simulink model "Final_project_template_R2020a_pt3 (1)"  (R2020a)
settings: Solver=FixedStepDiscrete  StartTime=0.0  StopTime=10.0  FixedStep=0.0005  RelTol=1e-3  EnableMultiTasking=on
InitFcn:
  | mbd_s32k_consistency_checks(bdroot(gcs));
values from neighbouring files (symbols this model uses):
  Ak = 100    [parameters_template (1).m]
  b = 100    [parameters_template (1).m]
  base_ids = [10, 20, 30, 40, 50, 70]    [parameters_template (1).m]
  dT = 0.01    [parameters_template (1).m]
  H = 20    [parameters_template (1).m]
  L1 = 1.6    [parameters_template (1).m]
  L2 = 0.8    [parameters_template (1).m]
  m = 2000    [parameters_template (1).m]
  n_desired = 2    [parameters_template (1).m]
  pot_gain = 1    [parameters_template (1).m]
  pot_offset = 512    [parameters_template (1).m]
  R = 1/5    (= 0.2)    [parameters_template (1).m]
  S_Kd1 = 0.03    [parameters_template (1).m]
  S_Kd2 = 25    [parameters_template (1).m]
  S_Kp1 = 0.45    [parameters_template (1).m]
  S_Kp2 = 1000    [parameters_template (1).m]
  V_Ki = 50    [parameters_template (1).m]
  V_Kp = 5000    [parameters_template (1).m]
undefined symbols (not defined in the file or in its folder): DiscIntNeverNeededParam, LQFP
libraries: mbd_s32k1xx_ec_toolbox x42, xpcutilitieslib x15, Veh_Sim x9, simulink x5
(part 2 of 2)

== system Final_project_template_R2020a_pt3 (1)/High Level Design/Outputs/Extract x,y,psi (Cars 1 - 6) ==
  s,n,psi,us (Cars 1 - 6) : Inport
  Demux : Demux  Outputs=6
  Extract x,y,psi : Subsystem
  Extract x,y,psi1 : Subsystem
  Extract x,y,psi2 : Subsystem
  Extract x,y,psi3 : Subsystem
  Extract x,y,psi4 : Subsystem
  Extract x,y,psi5 : Subsystem
  Mux : Mux  Inputs=6
  x,y,psi (Cars 1 - 6) : Outport  VectorParamsAs1DForOutWhenUnconnected=off
  wires:
  Demux/1 -> Extract x,y,psi/1(s,n,psi,us)
  Extract x,y,psi/1(x,y,psi) -> Mux/1
  Demux/2 -> Extract x,y,psi1/1(s,n,psi,us)
  Extract x,y,psi1/1(x,y,psi) -> Mux/2
  Demux/3 -> Extract x,y,psi2/1(s,n,psi,us)
  Extract x,y,psi2/1(x,y,psi) -> Mux/3
  Extract x,y,psi3/1(x,y,psi) -> Mux/4
  Demux/5 -> Extract x,y,psi4/1(s,n,psi,us)
  Extract x,y,psi4/1(x,y,psi) -> Mux/5
  s,n,psi,us (Cars 1 - 6)/1 -> Demux/1
  Extract x,y,psi5/1(x,y,psi) -> Mux/6
  Demux/6 -> Extract x,y,psi5/1(s,n,psi,us)
  Mux/1 -> x,y,psi (Cars 1 - 6)/1
  Demux/4 -> Extract x,y,psi3/1(s,n,psi,us)

== system Final_project_template_R2020a_pt3 (1)/High Level Design/Outputs/Tx CAN ==
  note: Use pack block to generate data arrays
      | Do not use any mailbox buffers that are used for receives
  note: Use FCAN_Send block to transmit two messages to the CAN bus
  s,n,psi,us : Inport
  "Byte Packing " : xpcutilitieslib/Byte Packing   MaskPackedDataType=uint8  MaskUnpackedDataTypes={'single'}  MaskAlignment=1
  Byte Packing 1 : xpcutilitieslib/Byte Packing   MaskPackedDataType=uint8  MaskUnpackedDataTypes={'single'}  MaskAlignment=1
  Constant : Constant  Value=8  OutDataTypeStr=uint8
  Constant1 : Constant  Value=8  OutDataTypeStr=uint8
  Demux : Demux  Outputs=2
  FCAN_Send : mbd_s32k1xx_ec_toolbox/Communication Blocks/CAN Blocks/FCAN_Send  can_instance=0  can_mode=Non-blocking  can_timeout_ms=0  can_mb_idx=0  can_extended_id=on  can_is_remote=off  can_id=41  show_adv_opts=off  can_fd_enable=off  can_enable_brs=off  can_fd_padding=0
  FCAN_Send1 : mbd_s32k1xx_ec_toolbox/Communication Blocks/CAN Blocks/FCAN_Send  can_instance=0  can_mode=Non-blocking  can_timeout_ms=0  can_mb_idx=1  can_extended_id=on  can_is_remote=off  can_id=42  show_adv_opts=off  can_fd_enable=off  can_enable_brs=off  can_fd_padding=0
  wires:
  s,n,psi,us/1 -> Demux/1
  Demux/1 -> "Byte Packing "/1
  Demux/2 -> Byte Packing 1/1
  "Byte Packing "/1 -> FCAN_Send/1
  Byte Packing 1/1 -> FCAN_Send1/1
  Constant1/1 -> FCAN_Send1/2
  Constant/1 -> FCAN_Send/2

== system Final_project_template_R2020a_pt3 (1)/High Level Design/Outputs/write torque ==
  Reaction Torque : Inport
  reaction torque : Subsystem
  wires:
  Reaction Torque/1 -> reaction torque/1(torque)

== system Final_project_template_R2020a_pt3 (1)/High Level Design/Vehicle Model/Phi dot ==
  delta : Inport
  u : Inport  Port=2
  Gain3 : Gain  Gain=1/L1
  Product1 : Product
  Trigonometric Function : Trigonometry
  Phi dot : Outport
  wires:
  Gain3/1 -> Product1/1
  Product1/1 -> Phi dot/1
  Trigonometric Function/1 -> Gain3/1
  u/1 -> Product1/2
  delta/1 -> Trigonometric Function/1

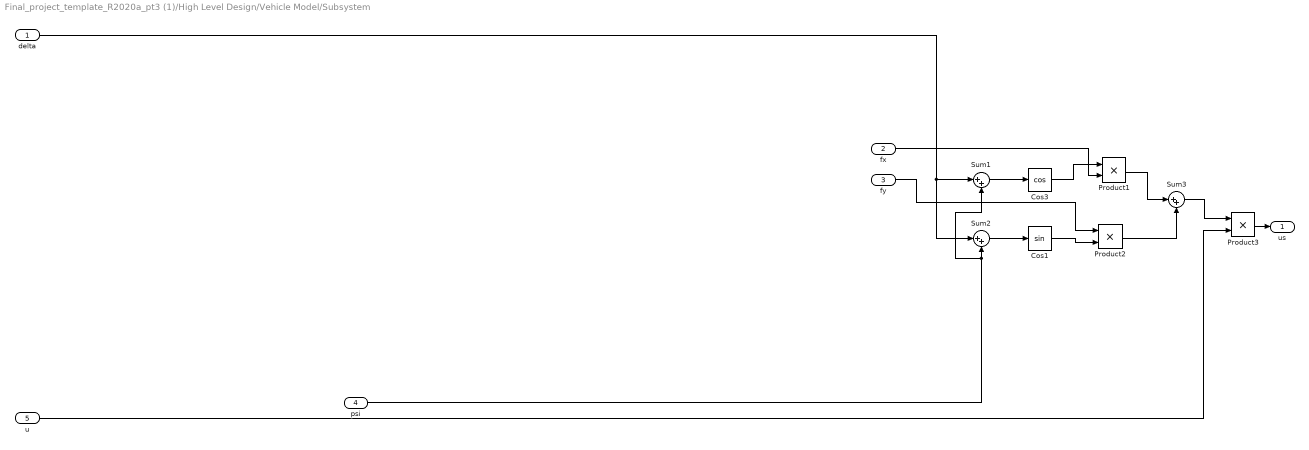
== system Final_project_template_R2020a_pt3 (1)/High Level Design/Vehicle Model/Subsystem ==
  delta : Inport
  fx : Inport  Port=2
  fy : Inport  Port=3
  psi : Inport  Port=4
  u : Inport  Port=5
  Cos1 : Trigonometry
  Cos3 : Trigonometry  Operator=cos
  Product1 : Product
  Product2 : Product
  Product3 : Product
  Sum1 : Sum  Inputs=|++
  Sum2 : Sum  Inputs=|++
  Sum3 : Sum  Inputs=|++
  us : Outport
  wires:
  Sum2/1 -> Cos1/1
  Cos3/1 -> Product1/1
  fy/1 -> Product2/1
  psi/1 -> Sum1/2, Sum2/2
  delta/1 -> Sum1/1, Sum2/1
  Product2/1 -> Sum3/2
  Sum3/1 -> Product3/1
  Product1/1 -> Sum3/1
  Cos1/1 -> Product2/2
  Sum1/1 -> Cos3/1
  fx/1 -> Product1/2
  Product3/1 -> us/1
  u/1 -> Product3/2

== system Final_project_template_R2020a_pt3 (1)/High Level Design/Vehicle Model/Subsystem1 ==
  Driving force (Fd) : Inport
  Discrete-Time Integrator : DiscreteIntegrator  SampleTime=-1  ICPrevOutput=DiscIntNeverNeededParam  ICPrevScaledInput=DiscIntNeverNeededParam
  Gain : Gain  Gain=1/m
  Gain1 : Gain  Gain=b
  Sum : Sum  Inputs=|+-
  u : Outport
  wires:
  Driving force (Fd)/1 -> Sum/1
  Gain1/1 -> Sum/2
  Gain/1 -> Discrete-Time Integrator/1
  Discrete-Time Integrator/1 -> u/1, Gain1/1
  Sum/1 -> Gain/1

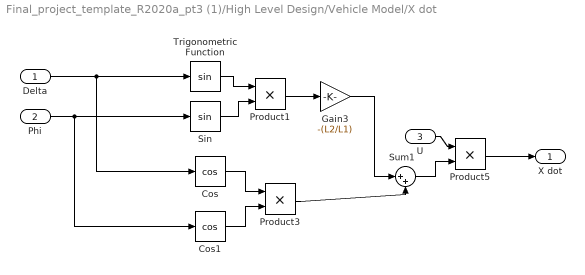
== system Final_project_template_R2020a_pt3 (1)/High Level Design/Vehicle Model/X dot  ==
  Delta : Inport
  Phi : Inport  Port=2
  U : Inport  Port=3
  Cos : Trigonometry  Operator=cos
  Cos1 : Trigonometry  Operator=cos
  Gain3 : Gain  Gain=-(L2/L1)
  Product1 : Product
  Product3 : Product
  Product5 : Product
  Sin : Trigonometry
  Sum1 : Sum  Inputs=|++
  Trigonometric Function : Trigonometry
  X dot : Outport
  wires:
  Sin/1 -> Product1/2
  Product1/1 -> Gain3/1
  Gain3/1 -> Sum1/1
  Trigonometric Function/1 -> Product1/1
  Sum1/1 -> Product5/2
  Product3/1 -> Sum1/2
  Delta/1 -> Cos/1, Trigonometric Function/1
  Cos/1 -> Product3/1
  Cos1/1 -> Product3/2
  Product5/1 -> X dot/1
  Phi/1 -> Cos1/1, Sin/1
  U/1 -> Product5/1

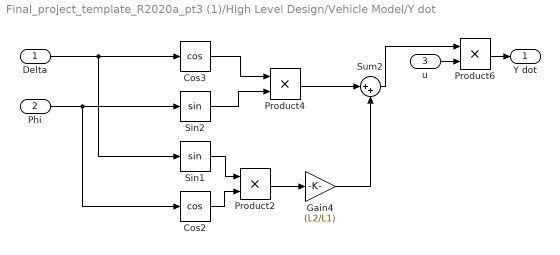
== system Final_project_template_R2020a_pt3 (1)/High Level Design/Vehicle Model/Y dot ==
  Delta : Inport
  Phi : Inport  Port=2
  u : Inport  Port=3
  Cos2 : Trigonometry  Operator=cos
  Cos3 : Trigonometry  Operator=cos
  Gain4 : Gain  Gain=(L2/L1)
  Product2 : Product
  Product4 : Product
  Product6 : Product
  Sin1 : Trigonometry
  Sin2 : Trigonometry
  Sum2 : Sum  Inputs=|++
  Y dot : Outport
  wires:
  Product4/1 -> Sum2/1
  Cos2/1 -> Product2/2
  Sin1/1 -> Product2/1
  Delta/1 -> Cos3/1, Sin1/1
  Sum2/1 -> Product6/1
  Gain4/1 -> Sum2/2
  Sin2/1 -> Product4/2
  Product2/1 -> Gain4/1
  Cos3/1 -> Product4/1
  Product6/1 -> Y dot/1
  u/1 -> Product6/2
  Phi/1 -> Cos2/1, Sin2/1

== system Final_project_template_R2020a_pt3 (1)/Serial Sim Out to Virtual Sim/UART Iteration/Resettable Subsystem ==
  Reset : ResetPort  DisableCoverage=on  ResetTriggerType=either
  Constant : Constant
  Delay : Delay  DelayLength=1
  Sum : Sum  Inputs=|++
  Out1 : Outport  VectorParamsAs1DForOutWhenUnconnected=off
  wires:
  Delay/1 -> Sum/1
  Constant/1 -> Sum/2
  Sum/1 -> Out1/1, Delay/1

== system Final_project_template_R2020a_pt3 (1)/Can Network Inputs/Extract CAN data/Data to s,n,psi,us /Switch Case Action Subsystem2 ==
  s,n : Inport
  Action Port : ActionPort  ActionPortLabel=if(u1 == 5)
  "Byte Unpacking " : xpcutilitieslib/Byte Unpacking   MaskUnpackedDataTypes={'single', 'single'}  MaskUnpackedDataSizes={[1], [1]}  MaskAlignment=1
      settings: SourceProductBaseCode=XP
  s : Outport  VectorParamsAs1DForOutWhenUnconnected=off
  n : Outport  Port=2  VectorParamsAs1DForOutWhenUnconnected=off
  wires:
  s,n/1 -> "Byte Unpacking "/1
  "Byte Unpacking "/1 -> s/1
  "Byte Unpacking "/2 -> n/1

== system Final_project_template_R2020a_pt3 (1)/Can Network Inputs/Extract CAN data/Data to s,n,psi,us /Switch Case Action Subsystem3 ==
  psi,us : Inport
  Action Port : ActionPort  ActionPortLabel=elseif(u1 == 6)
  "Byte Unpacking " : xpcutilitieslib/Byte Unpacking   MaskUnpackedDataTypes={'single', 'single'}  MaskUnpackedDataSizes={[1], [1]}  MaskAlignment=1
      settings: SourceProductBaseCode=XP
  psi : Outport  VectorParamsAs1DForOutWhenUnconnected=off
  us : Outport  Port=2  VectorParamsAs1DForOutWhenUnconnected=off
  wires:
  psi,us/1 -> "Byte Unpacking "/1
  "Byte Unpacking "/1 -> psi/1
  "Byte Unpacking "/2 -> us/1

== system Final_project_template_R2020a_pt3 (1)/Can Network Inputs/Extract CAN data/Data to s,n,psi,us 1/Switch Case Action Subsystem2 ==
  s,n : Inport
  Action Port : ActionPort  ActionPortLabel=if(u1 == 5)
  "Byte Unpacking " : xpcutilitieslib/Byte Unpacking   MaskUnpackedDataTypes={'single', 'single'}  MaskUnpackedDataSizes={[1], [1]}  MaskAlignment=1
      settings: SourceProductBaseCode=XP
  s : Outport  VectorParamsAs1DForOutWhenUnconnected=off
  n : Outport  Port=2  VectorParamsAs1DForOutWhenUnconnected=off
  wires:
  s,n/1 -> "Byte Unpacking "/1
  "Byte Unpacking "/1 -> s/1
  "Byte Unpacking "/2 -> n/1

== system Final_project_template_R2020a_pt3 (1)/Can Network Inputs/Extract CAN data/Data to s,n,psi,us 1/Switch Case Action Subsystem3 ==
  psi,us : Inport
  Action Port : ActionPort  ActionPortLabel=elseif(u1 == 6)
  "Byte Unpacking " : xpcutilitieslib/Byte Unpacking   MaskUnpackedDataTypes={'single', 'single'}  MaskUnpackedDataSizes={[1], [1]}  MaskAlignment=1
      settings: SourceProductBaseCode=XP
  psi : Outport  VectorParamsAs1DForOutWhenUnconnected=off
  us : Outport  Port=2  VectorParamsAs1DForOutWhenUnconnected=off
  wires:
  psi,us/1 -> "Byte Unpacking "/1
  "Byte Unpacking "/1 -> psi/1
  "Byte Unpacking "/2 -> us/1

== system Final_project_template_R2020a_pt3 (1)/Can Network Inputs/Extract CAN data/Data to s,n,psi,us 2/Switch Case Action Subsystem2 ==
  s,n : Inport
  Action Port : ActionPort  ActionPortLabel=if(u1 == 5)
  "Byte Unpacking " : xpcutilitieslib/Byte Unpacking   MaskUnpackedDataTypes={'single', 'single'}  MaskUnpackedDataSizes={[1], [1]}  MaskAlignment=1
      settings: SourceProductBaseCode=XP
  s : Outport  VectorParamsAs1DForOutWhenUnconnected=off
  n : Outport  Port=2  VectorParamsAs1DForOutWhenUnconnected=off
  wires:
  s,n/1 -> "Byte Unpacking "/1
  "Byte Unpacking "/1 -> s/1
  "Byte Unpacking "/2 -> n/1

== system Final_project_template_R2020a_pt3 (1)/Can Network Inputs/Extract CAN data/Data to s,n,psi,us 2/Switch Case Action Subsystem3 ==
  psi,us : Inport
  Action Port : ActionPort  ActionPortLabel=elseif(u1 == 6)
  "Byte Unpacking " : xpcutilitieslib/Byte Unpacking   MaskUnpackedDataTypes={'single', 'single'}  MaskUnpackedDataSizes={[1], [1]}  MaskAlignment=1
      settings: SourceProductBaseCode=XP
  psi : Outport  VectorParamsAs1DForOutWhenUnconnected=off
  us : Outport  Port=2  VectorParamsAs1DForOutWhenUnconnected=off
  wires:
  psi,us/1 -> "Byte Unpacking "/1
  "Byte Unpacking "/1 -> psi/1
  "Byte Unpacking "/2 -> us/1

== system Final_project_template_R2020a_pt3 (1)/Can Network Inputs/Extract CAN data/Data to s,n,psi,us 3/Switch Case Action Subsystem2 ==
  s,n : Inport
  Action Port : ActionPort  ActionPortLabel=if(u1 == 5)
  "Byte Unpacking " : xpcutilitieslib/Byte Unpacking   MaskUnpackedDataTypes={'single', 'single'}  MaskUnpackedDataSizes={[1], [1]}  MaskAlignment=1
      settings: SourceProductBaseCode=XP
  s : Outport  VectorParamsAs1DForOutWhenUnconnected=off
  n : Outport  Port=2  VectorParamsAs1DForOutWhenUnconnected=off
  wires:
  s,n/1 -> "Byte Unpacking "/1
  "Byte Unpacking "/1 -> s/1
  "Byte Unpacking "/2 -> n/1

== system Final_project_template_R2020a_pt3 (1)/Can Network Inputs/Extract CAN data/Data to s,n,psi,us 3/Switch Case Action Subsystem3 ==
  psi,us : Inport
  Action Port : ActionPort  ActionPortLabel=elseif(u1 == 6)
  "Byte Unpacking " : xpcutilitieslib/Byte Unpacking   MaskUnpackedDataTypes={'single', 'single'}  MaskUnpackedDataSizes={[1], [1]}  MaskAlignment=1
      settings: SourceProductBaseCode=XP
  psi : Outport  VectorParamsAs1DForOutWhenUnconnected=off
  us : Outport  Port=2  VectorParamsAs1DForOutWhenUnconnected=off
  wires:
  psi,us/1 -> "Byte Unpacking "/1
  "Byte Unpacking "/1 -> psi/1
  "Byte Unpacking "/2 -> us/1

== system Final_project_template_R2020a_pt3 (1)/Can Network Inputs/Extract CAN data/Data to s,n,psi,us 4/Switch Case Action Subsystem2 ==
  s,n : Inport
  Action Port : ActionPort  ActionPortLabel=if(u1 == 5)
  "Byte Unpacking " : xpcutilitieslib/Byte Unpacking   MaskUnpackedDataTypes={'single', 'single'}  MaskUnpackedDataSizes={[1], [1]}  MaskAlignment=1
      settings: SourceProductBaseCode=XP
  s : Outport  VectorParamsAs1DForOutWhenUnconnected=off
  n : Outport  Port=2  VectorParamsAs1DForOutWhenUnconnected=off
  wires:
  s,n/1 -> "Byte Unpacking "/1
  "Byte Unpacking "/1 -> s/1
  "Byte Unpacking "/2 -> n/1

== system Final_project_template_R2020a_pt3 (1)/Can Network Inputs/Extract CAN data/Data to s,n,psi,us 4/Switch Case Action Subsystem3 ==
  psi,us : Inport
  Action Port : ActionPort  ActionPortLabel=elseif(u1 == 6)
  "Byte Unpacking " : xpcutilitieslib/Byte Unpacking   MaskUnpackedDataTypes={'single', 'single'}  MaskUnpackedDataSizes={[1], [1]}  MaskAlignment=1
      settings: SourceProductBaseCode=XP
  psi : Outport  VectorParamsAs1DForOutWhenUnconnected=off
  us : Outport  Port=2  VectorParamsAs1DForOutWhenUnconnected=off
  wires:
  psi,us/1 -> "Byte Unpacking "/1
  "Byte Unpacking "/1 -> psi/1
  "Byte Unpacking "/2 -> us/1

== system Final_project_template_R2020a_pt3 (1)/Can Network Inputs/Extract CAN data/Data to s,n,psi,us 5/Switch Case Action Subsystem2 ==
  s,n : Inport
  Action Port : ActionPort  ActionPortLabel=if(u1 == 5)
  "Byte Unpacking " : xpcutilitieslib/Byte Unpacking   MaskUnpackedDataTypes={'single', 'single'}  MaskUnpackedDataSizes={[1], [1]}  MaskAlignment=1
      settings: SourceProductBaseCode=XP
  s : Outport  VectorParamsAs1DForOutWhenUnconnected=off
  n : Outport  Port=2  VectorParamsAs1DForOutWhenUnconnected=off
  wires:
  s,n/1 -> "Byte Unpacking "/1
  "Byte Unpacking "/1 -> s/1
  "Byte Unpacking "/2 -> n/1

== system Final_project_template_R2020a_pt3 (1)/Can Network Inputs/Extract CAN data/Data to s,n,psi,us 5/Switch Case Action Subsystem3 ==
  psi,us : Inport
  Action Port : ActionPort  ActionPortLabel=elseif(u1 == 6)
  "Byte Unpacking " : xpcutilitieslib/Byte Unpacking   MaskUnpackedDataTypes={'single', 'single'}  MaskUnpackedDataSizes={[1], [1]}  MaskAlignment=1
      settings: SourceProductBaseCode=XP
  psi : Outport  VectorParamsAs1DForOutWhenUnconnected=off
  us : Outport  Port=2  VectorParamsAs1DForOutWhenUnconnected=off
  wires:
  psi,us/1 -> "Byte Unpacking "/1
  "Byte Unpacking "/1 -> psi/1
  "Byte Unpacking "/2 -> us/1

== system Final_project_template_R2020a_pt3 (1)/High Level Design/Auto Cruise Control/ACC State Logic/Subsystem ==
  us : Inport
  usi : Inport  Port=2
  si : Inport  Port=3
  s : Inport  Port=4
  Enable : EnablePort
  Constant : Constant  Value=H
  En_choice : Stateflow chart  TreatAsAtomicUnit=on
  en_vel : Outport
  en_pos : Outport  Port=2
  wires:
  s/1 -> En_choice/5(Sm)
  usi/1 -> En_choice/1(Usi)
  us/1 -> En_choice/2(Us)
  si/1 -> En_choice/4(Si)
  Constant/1 -> En_choice/3(H)
  En_choice/1(en_vel) -> en_vel/1
  En_choice/2(en_pos) -> en_pos/1

== system Final_project_template_R2020a_pt3 (1)/High Level Design/Auto Cruise Control/Speed Ctrl/PI ==
  Error : Inport
  Gain : Gain  Gain=V_Ki  SaturateOnIntegerOverflow=on  OutDataTypeStr=Inherit: Same as input  ParamDataTypeStr=Inherit: Same as input
  Gain1 : Gain  Gain=V_Kp  SaturateOnIntegerOverflow=on  OutDataTypeStr=Inherit: Same as input  ParamDataTypeStr=Inherit: Same as input
  My Discrete Integrator : Subsystem
  Sum : Sum  Inputs=|++  SaturateOnIntegerOverflow=on
  U : Outport
  wires:
  Sum/1 -> U/1
  Error/1 -> Gain1/1, Gain/1
  Gain1/1 -> Sum/2
  My Discrete Integrator/1(X) -> Sum/1
  Gain/1 -> My Discrete Integrator/1(X_dot)

== system Final_project_template_R2020a_pt3 (1)/High Level Design/Inputs/get wheel position/count to radians ==
  In1 : Inport
  Data Type Conversion : DataTypeConversion  OutDataTypeStr=uint16
  Data Type Conversion1 : DataTypeConversion  OutDataTypeStr=int16
  Data Type Conversion2 : DataTypeConversion  OutDataTypeStr=single
  Gain : Gain  Gain=360/4000
  Gain1 : Gain  Gain=(2*pi)/360
  Sum : Sum  Inputs=|+-
  Sum1 : Sum  Inputs=|++
  Unit Delay : UnitDelay  SampleTime=-1  HasFrameUpgradeWarning=on
  Unit Delay1 : UnitDelay  SampleTime=-1  HasFrameUpgradeWarning=on
  Haptic Wheel Position (radians) : Outport
  wires:
  Data Type Conversion2/1 -> Gain/1
  Sum/1 -> Data Type Conversion1/1
  Data Type Conversion/1 -> Unit Delay/1, Sum/1
  Unit Delay/1 -> Sum/2
  Sum1/1 -> Gain1/1, Unit Delay1/1
  Data Type Conversion1/1 -> Data Type Conversion2/1
  Unit Delay1/1 -> Sum1/2
  Gain/1 -> Sum1/1
  In1/1 -> Data Type Conversion/1
  Gain1/1 -> Haptic Wheel Position (radians)/1

== system Final_project_template_R2020a_pt3 (1)/High Level Design/Outputs/Extract x,y,psi (Cars 1 - 6)/Extract x,y,psi ==
  s,n,psi,us : Inport
  Demux : Demux
  Mux : Mux  Inputs=3
  Terminator : Terminator
  s,n to x,y : Veh_Sim/s,n to x,y  SystemSampleTime=-1  Latency=0  AutoFrameSizeCalculation=off
  x,y,psi : Outport  VectorParamsAs1DForOutWhenUnconnected=off
  wires:
  Demux/1 -> s,n to x,y/1
  Demux/2 -> s,n to x,y/2
  s,n,psi,us/1 -> Demux/1
  s,n to x,y/1 -> Mux/1
  s,n to x,y/2 -> Mux/2
  Demux/3 -> Mux/3
  Mux/1 -> x,y,psi/1
  Demux/4 -> Terminator/1

== system Final_project_template_R2020a_pt3 (1)/High Level Design/Outputs/Extract x,y,psi (Cars 1 - 6)/Extract x,y,psi1 ==
  s,n,psi,us : Inport
  Demux : Demux
  Mux : Mux  Inputs=3
  Terminator : Terminator
  s,n to x,y : Veh_Sim/s,n to x,y  SystemSampleTime=-1  Latency=0  AutoFrameSizeCalculation=off
  x,y,psi : Outport  VectorParamsAs1DForOutWhenUnconnected=off
  wires:
  Demux/1 -> s,n to x,y/1
  Demux/2 -> s,n to x,y/2
  s,n,psi,us/1 -> Demux/1
  s,n to x,y/1 -> Mux/1
  s,n to x,y/2 -> Mux/2
  Demux/3 -> Mux/3
  Mux/1 -> x,y,psi/1
  Demux/4 -> Terminator/1

== system Final_project_template_R2020a_pt3 (1)/High Level Design/Outputs/Extract x,y,psi (Cars 1 - 6)/Extract x,y,psi2 ==
  s,n,psi,us : Inport
  Demux : Demux
  Mux : Mux  Inputs=3
  Terminator : Terminator
  s,n to x,y : Veh_Sim/s,n to x,y  SystemSampleTime=-1  Latency=0  AutoFrameSizeCalculation=off
  x,y,psi : Outport  VectorParamsAs1DForOutWhenUnconnected=off
  wires:
  Demux/1 -> s,n to x,y/1
  Demux/2 -> s,n to x,y/2
  s,n,psi,us/1 -> Demux/1
  s,n to x,y/1 -> Mux/1
  s,n to x,y/2 -> Mux/2
  Demux/3 -> Mux/3
  Mux/1 -> x,y,psi/1
  Demux/4 -> Terminator/1

== system Final_project_template_R2020a_pt3 (1)/High Level Design/Outputs/Extract x,y,psi (Cars 1 - 6)/Extract x,y,psi3 ==
  s,n,psi,us : Inport
  Demux : Demux
  Mux : Mux  Inputs=3
  Terminator : Terminator
  s,n to x,y : Veh_Sim/s,n to x,y  SystemSampleTime=-1  Latency=0  AutoFrameSizeCalculation=off
  x,y,psi : Outport  VectorParamsAs1DForOutWhenUnconnected=off
  wires:
  Demux/1 -> s,n to x,y/1
  Demux/2 -> s,n to x,y/2
  s,n,psi,us/1 -> Demux/1
  s,n to x,y/1 -> Mux/1
  s,n to x,y/2 -> Mux/2
  Demux/3 -> Mux/3
  Mux/1 -> x,y,psi/1
  Demux/4 -> Terminator/1

== system Final_project_template_R2020a_pt3 (1)/High Level Design/Outputs/Extract x,y,psi (Cars 1 - 6)/Extract x,y,psi4 ==
  s,n,psi,us : Inport
  Demux : Demux
  Mux : Mux  Inputs=3
  Terminator : Terminator
  s,n to x,y : Veh_Sim/s,n to x,y  SystemSampleTime=-1  Latency=0  AutoFrameSizeCalculation=off
  x,y,psi : Outport  VectorParamsAs1DForOutWhenUnconnected=off
  wires:
  Demux/1 -> s,n to x,y/1
  Demux/2 -> s,n to x,y/2
  s,n,psi,us/1 -> Demux/1
  s,n to x,y/1 -> Mux/1
  s,n to x,y/2 -> Mux/2
  Demux/3 -> Mux/3
  Mux/1 -> x,y,psi/1
  Demux/4 -> Terminator/1

== system Final_project_template_R2020a_pt3 (1)/High Level Design/Outputs/Extract x,y,psi (Cars 1 - 6)/Extract x,y,psi5 ==
  s,n,psi,us : Inport
  Demux : Demux
  Mux : Mux  Inputs=3
  Terminator : Terminator
  s,n to x,y : Veh_Sim/s,n to x,y  SystemSampleTime=-1  Latency=0  AutoFrameSizeCalculation=off
  x,y,psi : Outport  VectorParamsAs1DForOutWhenUnconnected=off
  wires:
  Demux/1 -> s,n to x,y/1
  Demux/2 -> s,n to x,y/2
  s,n,psi,us/1 -> Demux/1
  s,n to x,y/1 -> Mux/1
  s,n to x,y/2 -> Mux/2
  Demux/3 -> Mux/3
  Mux/1 -> x,y,psi/1
  Demux/4 -> Terminator/1

== system Final_project_template_R2020a_pt3 (1)/High Level Design/Outputs/write torque/reaction torque ==
  torque : Inport
  Constant : Constant  Value=0.5  OutDataTypeStr=single
  FTM_PWM_Config : mbd_s32k1xx_ec_toolbox/Motor Control Blocks/FTM Blocks/FTM_PWM_Config  ftmModule=0  ftmMode=Edge-Aligned PWM  ftmSourceClock=80 MHz  swcontrol_enable=off  chan0En=on  chan0Type=Complementary  chan2En=off  chan2Type=Independent  chan4En=off  chan4Type=Independent  chan6En=off  chan6Type=Independent  ftmPwmUnits=Hz  outFrequency=20000  ftmPeriod=4000  ftmPrescaler=Divide by 1  deadtimeUnits=Nanoseconds  deadtimeNs=0  deadtimeTicks=0  deadtimePrescaler=Divide by 1  dutyCycleCh0=0.25  dutyCycleCh1=0.25  dutyCycleCh2=0.25  dutyCycleCh3=0.25  dutyCycleCh4=0.25  dutyCycleCh5=0.25  dutyCycleCh6=0.25  dutyCycleCh7=0.25  dutyCycleSim=on  startAfterInit=on  showAdvOpt=on  pinFtmCh0=PTB12: [FTM0_CH0 | FTM Channel]  pinFtmCh1=None  pinPolCh0=Active Low  pinPolCh1=Active Low  outputComplem0=Main duplicated  outputLevel0=Low  outputLevel1=Low  pinFtmCh2=PTC2: [FTM0_CH2 | FTM Channel]  pinFtmCh3=None  pinPolCh2=Active Low  pinPolCh3=Active Low  outputComplem2=Main duplicated  outputLevel2=Low  outputLevel3=Low  pinFtmCh4=PTB4: [FTM0_CH4 | FTM Channel]  pinFtmCh5=None  pinPolCh4=Active Low  pinPolCh5=Active Low  outputComplem4=Main duplicated  outputLevel4=Low  outputLevel5=Low  pinFtmCh6=PTA17: [FTM0_CH6 | FTM Channel]  pinFtmCh7=None  pinPolCh6=Active Low  pinPolCh7=Active Low  outputComplem6=Main duplicated  outputLevel6=Low  outputLevel7=Low  initTrigger=off  chTrigger0=off  chTrigger1=off  chTrigger2=off  chTrigger3=off  chTrigger4=off  chTrigger5=off  chTrigger6=off  chTrigger7=off  mcuTargetUpdate=on  pwmSyncTrg=Software trigger  pwmSyncHwRouting=TRGMUX_FTM7  pwmSyncTrg0=off  pwmSyncTrg1=off  pwmSyncTrg2=off  pwmSyncAutoClear=on  pwmSyncMinLoad=on  pwmSyncMaxLoad=on  pwmSyncInvert=System Clock  pwmSyncOutControl=System Clock  pwmSyncOutMask=System Clock  pwmSyncCounterInitial=System Clock  pwmSyncPoints=Update now  reloadEnable=off  reloadPriority=15  reloadHalfCycle=off  reloadHCR=0  reloadFrequency=0  chnMatch0=off  chnMatch1=off  chnMatch2=off  chnMatch3=off  chnMatch4=off  chnMatch5=off  chnMatch6=off  chnMatch7=off  pwmFaultProtection=off  pwmFaultInterrupt=off  pwmFaultClearing=Fault control disabled  pwmFaultPinState=Safe Value  pwmFaultFilterValue=0  pwmFaultPriority=15  fault_disen_0=off  fault_filter_0=off  fault_polarity_0=Active High  fault_disen_1=off  fault_filter_1=off  fault_polarity_1=Active high  fault_disen_2=off  fault_filter_2=off  fault_polarity_2=Active high  fault_disen_3=off  fault_filter_3=off  fault_polarity_3=Active high  fault_pin_0=None  fault_pin_1=None  fault_pin_2=None  fault_pin_3=None
  Gain : Gain  Gain=3.16e-4
  Saturation : Saturate  UpperLimit=0.76  LowerLimit=0.24
  Sum : Sum  Inputs=|++  OutDataTypeStr=single
  Terminator : Terminator
  wires:
  Saturation/1 -> FTM_PWM_Config/1
  torque/1 -> Gain/1
  FTM_PWM_Config/1 -> Terminator/1
  Gain/1 -> Sum/1
  Constant/1 -> Sum/2
  Sum/1 -> Saturation/1

== system Final_project_template_R2020a_pt3 (1)/High Level Design/Auto Cruise Control/Speed Ctrl/PI/My Discrete Integrator ==
  X_dot : Inport
  Gain : Gain  Gain=dT  SaturateOnIntegerOverflow=on  OutDataTypeStr=Inherit: Same as input  ParamDataTypeStr=Inherit: Same as input
  Sum : Sum  Inputs=|++  InputSameDT=on  SaturateOnIntegerOverflow=on  OutDataTypeStr=Inherit: Same as first input
  Unit Delay : UnitDelay  SampleTime=-1  HasFrameUpgradeWarning=on
  X : Outport
  wires:
  Gain/1 -> Sum/1
  X_dot/1 -> Gain/1
  Sum/1 -> Unit Delay/1
  Unit Delay/1 -> Sum/2, X/1

== matlab function Final_project_template_R2020a_pt3 (1)/High Level Design/Auto Cruise Control/ACC State Logic/MATLAB Function ==
  data: s_all input; si output; i output
function [si, i] = fcn(s_all)
    i = 1;
    s_mycar=s_all(1);
    
    mindist = single(99999);
    for idx=2:7
        dist = s_all(idx) - s_mycar;
        if dist > 0 && s_all(idx) < mindist
            i = idx;
            mindist = s_all(idx);
        end
    end
    if(mindist == single(99999))
        mindist = s_all(1);
    end
    si = mindist;
end

== stateflow chart Final_project_template_R2020a_pt3 (1)/High Level Design/Auto Cruise Control/ACC State Logic/Subsystem/En_choice ==
  state PositionControl_
    en_vel = false;
    en_pos = true;
  state VelocityControl_
    en_vel = true;
    en_pos = false;
  PositionControl_ -> VelocityControl_ : [(Usi>Us) || (Si-Sm>H)]
  (default) -> VelocityControl_
  VelocityControl_ -> PositionControl_ : [(Usi<Us) && (Si-Sm<=H)]
  data: en_vel output boolean; en_pos output boolean; Usi input; Us input; H input; Si input; Sm input
